simulink model "Vertical_System_Control_PID"  (R2014a)
settings: Solver=ode45  StartTime=0.0  StopTime=20  RelTol=1e-3
libraries: simulink x2
settings Model: Creator=pmdbpc  LastModifiedBy=pmdbpc

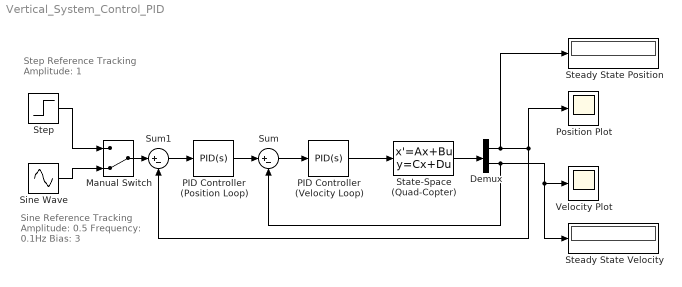
== system Vertical_System_Control_PID ==
  note: Sine Reference Tracking
      | Amplitude: 0.5
      | Frequency: 0.1Hz
      | Bias: 3
  note: Step Reference Tracking
      | Amplitude: 1
  Demux : Demux  Outputs=2
  Manual Switch : ManualSwitch  CurrentSetting=0
  PID Controller (Position Loop) : simulink/Continuous/PID Controller  Controller=PID  TimeDomain=Continuous-time  SampleTime=1  IntegratorMethod=Forward Euler  FilterMethod=Forward Euler  Form=Parallel  P=1.4420202461893  I=0.0165472199278363  D=3.45017715727879  N=2.86528364104348  InitialConditionSource=internal  InitialConditionForIntegrator=0  InitialConditionForFilter=0  ExternalReset=none  LimitOutput=off  UpperSaturationLimit=inf  LowerSaturationLimit=-inf  LinearizeAsGain=on  AntiWindupMode=none  Kb=1  TrackingMode=off  Kt=1  PParamMin=[]  PParamMax=[]  IParamMin=[]  IParamMax=[]  DParamMin=[]  DParamMax=[]  NParamMin=[]  NParamMax=[]  KbParamMin=[]  KbParamMax=[]  KtParamMin=[]  KtParamMax=[]  POutMin=[]  POutMax=[]  IOutMin=[]  IOutMax=[]  DOutMin=[]  DOutMax=[]  NOutMin=[]  NOutMax=[]  KbOutMin=[]  KbOutMax=[]  KtOutMin=[]  KtOutMax=[]  IntegratorOutMin=[]  IntegratorOutMax=[]  FilterOutMin=[]  FilterOutMax=[]  SumOutMin=[]  SumOutMax=[]  SumI1OutMin=[]  SumI1OutMax=[]  SumI2OutMin=[]  SumI2OutMax=[]  SumI3OutMin=[]  SumI3OutMax=[]  SumDOutMin=[]  SumDOutMax=[]  SaturationOutMin=[]  SaturationOutMax=[]  IntegratorContinuousStateAttributes=''  IntegratorStateMustResolveToSignalObject=off  IntegratorRTWStateStorageClass=Auto  FilterContinuousStateAttributes=''  FilterStateMustResolveToSignalObject=off  FilterRTWStateStorageClass=Auto
  PID Controller (Velocity Loop) : simulink/Continuous/PID Controller  Controller=PID  TimeDomain=Continuous-time  SampleTime=1  IntegratorMethod=Forward Euler  FilterMethod=Forward Euler  Form=Parallel  P=-12.6851452532975  I=-0.330034251333615  D=-1.07766572687637  N=340.555964750453  InitialConditionSource=internal  InitialConditionForIntegrator=0  InitialConditionForFilter=0  ExternalReset=none  LimitOutput=off  UpperSaturationLimit=inf  LowerSaturationLimit=-inf  LinearizeAsGain=on  AntiWindupMode=none  Kb=1  TrackingMode=off  Kt=1  PParamMin=[]  PParamMax=[]  IParamMin=[]  IParamMax=[]  DParamMin=[]  DParamMax=[]  NParamMin=[]  NParamMax=[]  KbParamMin=[]  KbParamMax=[]  KtParamMin=[]  KtParamMax=[]  POutMin=[]  POutMax=[]  IOutMin=[]  IOutMax=[]  DOutMin=[]  DOutMax=[]  NOutMin=[]  NOutMax=[]  KbOutMin=[]  KbOutMax=[]  KtOutMin=[]  KtOutMax=[]  IntegratorOutMin=[]  IntegratorOutMax=[]  FilterOutMin=[]  FilterOutMax=[]  SumOutMin=[]  SumOutMax=[]  SumI1OutMin=[]  SumI1OutMax=[]  SumI2OutMin=[]  SumI2OutMax=[]  SumI3OutMin=[]  SumI3OutMax=[]  SumDOutMin=[]  SumDOutMax=[]  SaturationOutMin=[]  SaturationOutMax=[]  IntegratorContinuousStateAttributes=''  IntegratorStateMustResolveToSignalObject=off  IntegratorRTWStateStorageClass=Auto  FilterContinuousStateAttributes=''  FilterStateMustResolveToSignalObject=off  FilterRTWStateStorageClass=Auto
  Position Plot : Scope
      settings: SaveName=P_Ctrlr_Pos_PID
  Sine Wave : Sin  Amplitude=0.5  Bias=3  Frequency=0.1*6.28  SampleTime=0
  State-Space (Quad-Copter) : StateSpace  A=[0 1 0 0 0 0; 0 0 -0.0106 0.0106 -0.0106 0.0106; 0 0 -10 0 0 0; 0 0 0 -10 0 0; 0 0 0 0 -10 0; 0 0 0 0 0 -10]  B=[0; 0; 7; -7; 7; -7]  C=[1 0 0 0 0 0; 0 1 0 0 0 0]  D=[0; 0]  X0=[5 0 0 0 0 0]  ContinuousStateAttributes={'z','w','o1','o2','o3','o4'}
  Steady State Position : Display
  Steady State Velocity : Display
  Step : Step  Time=0  SampleTime=0.001
  Sum : Sum  Inputs=|+-
  Sum1 : Sum  Inputs=|+-
  Velocity Plot : Scope
      settings: SaveName=P_Ctrlr_Speed_PID
  wires:
  Step/1 -> Manual Switch/1
  State-Space (Quad-Copter)/1 -> Demux/1
  Demux/2 -> Velocity Plot/1, Steady State Velocity/1, Sum/2
  PID Controller (Velocity Loop)/1 -> State-Space (Quad-Copter)/1
  Sum/1 -> PID Controller (Velocity Loop)/1
  Sum1/1 -> PID Controller (Position Loop)/1
  PID Controller (Position Loop)/1 -> Sum/1
  Demux/1 -> Position Plot/1, Sum1/2, Steady State Position/1
  Manual Switch/1 -> Sum1/1
  Sine Wave/1 -> Manual Switch/2
